simulink model "KalmanFilterHeli"  (R2021a)
settings: Solver=VariableStepAuto  StartTime=0.0  StopTime=10.0  MaxStep=1e-3  RelTol=1e-3
values from neighbouring files (symbols this model uses):
  A = [0 0 1 0 ... (first row only)    [HeliControlGain.m]    (also in HeliControlHinf.m; HeliControlInteger.m; HeliControlLQG.m; HeliControlLQRgain.m)
  Afk = A-L*C    [HeliControlLQG.m]
  B = [0 0 ... (first row only)    [HeliControlGain.m]    (also in HeliControlHinf.m; HeliControlInteger.m; HeliControlLQG.m; HeliControlLQRgain.m)
  Bfk = [B-L*D L]    [HeliControlLQG.m]
  C = [1 0 0 0 ... (first row only)    [HeliControlGain.m]    (also in HeliControlHinf.m; HeliControlInteger.m; HeliControlLQG.m; HeliControlLQRgain.m)
  Cfk = eye(4)    [HeliControlLQG.m]
  D = zeros(2,2)    [HeliControlGain.m]    (also in HeliControlHinf.m; HeliControlInteger.m; HeliControlLQG.m; HeliControlLQRgain.m)
  Dfk = zeros(4,4)    [HeliControlLQG.m]
  Kf = K(:,1:4)    [HeliControlInteger.m]    (also in HeliControlIntegerObsv.m; HeliControlLQG.m; HeliControlLQRinteger.m)
  Ki = K(:,5:end)    [HeliControlInteger.m]    (also in HeliControlIntegerObsv.m; HeliControlLQG.m; HeliControlLQRinteger.m)
  Qtilde = v_x*diag([1 1 1 1])    [HeliControlLQG.m]
  Rtilde = v_y*diag([1 1])    [HeliControlLQG.m]
  T = feedback(L,eye(2))    [HeliControlHinf.m]    (also in HeliControlLQG.m = 0.00333333333333)
libraries: simulink x2
settings Model: Creator=Ciro  LastModifiedBy=Ciro

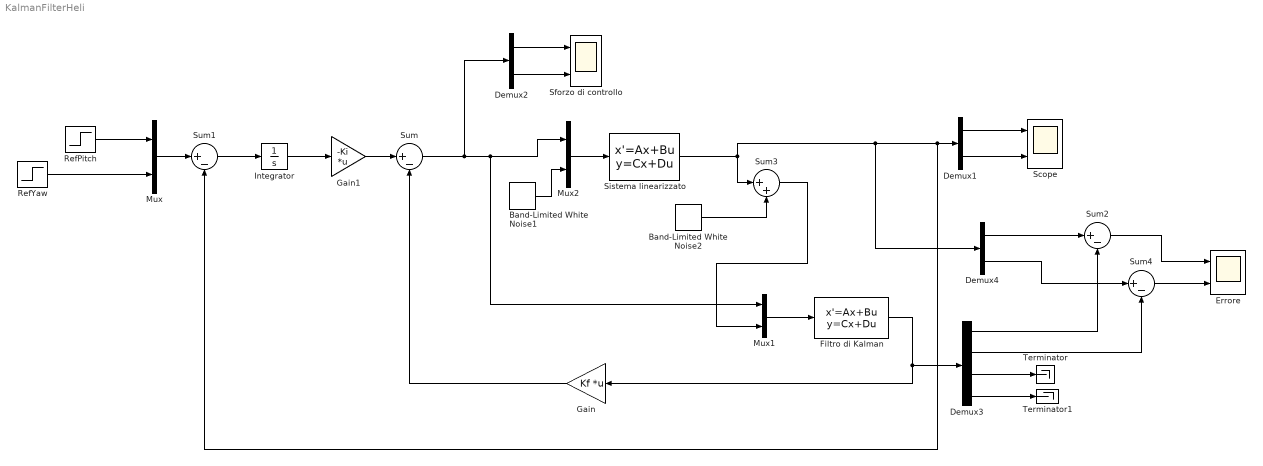
== system KalmanFilterHeli ==
  Band-Limited White Noise1 : simulink/Sources/Band-Limited White Noise  Cov=diag(Qtilde)  Ts=T  seed=[23341]
  Band-Limited White Noise2 : simulink/Sources/Band-Limited White Noise  Cov=diag(Rtilde)  Ts=T  seed=[23341]
  Demux1 : Demux  Outputs=2
  Demux2 : Demux  Outputs=2
  Demux3 : Demux
  Demux4 : Demux  Outputs=2
  Errore : Scope  NumInputPorts=2
  Filtro di Kalman : StateSpace  A=Afk  B=Bfk  C=Cfk  D=Dfk  InitialCondition=0
  Gain : Gain  Gain=Kf  Multiplication=Matrix(K*u)
  Gain1 : Gain  Gain=-Ki  Multiplication=Matrix(K*u)
  Integrator : Integrator
  Mux : Mux  Inputs=2
  Mux1 : Mux  Inputs=2
  Mux2 : Mux  Inputs=2
  RefPitch : Step  After=0.3  SampleTime=0
  RefYaw : Step  After=0.3  SampleTime=0
  Scope : Scope  NumInputPorts=2
  Sforzo di controllo : Scope  NumInputPorts=2
  Sistema linearizzato : StateSpace  A=A  B=[B eye(4)]  C=C  D=[D zeros(2,4)]  InitialCondition=[0;0;0;0]  ParameterTunability=Optimized
  Sum{,1..2,4} (4 alike) : Sum  Inputs=|+-
  Sum3 : Sum  Inputs=|++
  Terminator : Terminator
  Terminator1 : Terminator
  wires:
  Demux1/1 -> Scope/1
  Demux2/2 -> Sforzo di controllo/2
  Demux1/2 -> Scope/2
  Integrator/1 -> Gain1/1
  Sum/1 -> Demux2/1, Mux1/1, Mux2/1
  Mux2/1 -> Sistema linearizzato/1
  Mux/1 -> Sum1/1
  Sum1/1 -> Integrator/1
  RefYaw/1 -> Mux/2
  RefPitch/1 -> Mux/1
  Gain/1 -> Sum/2
  Gain1/1 -> Sum/1
  Demux2/1 -> Sforzo di controllo/1
  Filtro di Kalman/1 -> Gain/1, Demux3/1
  Mux1/1 -> Filtro di Kalman/1
  Band-Limited White Noise1/1 -> Mux2/2
  Band-Limited White Noise2/1 -> Sum3/2
  Sum3/1 -> Mux1/2
  Sistema linearizzato/1 -> Demux4/1, Sum1/2, Demux1/1, Sum3/1
  Demux3/3 -> Terminator/1
  Demux3/4 -> Terminator1/1
  Demux4/1 -> Sum2/1
  Demux3/1 -> Sum2/2
  Sum2/1 -> Errore/1
  Demux4/2 -> Sum4/1
  Demux3/2 -> Sum4/2
  Sum4/1 -> Errore/2
